simulink model "simpleModel"  (R2014b)
settings: Solver=ode45  StartTime=0.0  StopTime=10.0  RelTol=1e-3
settings Model: Creator=dmeissne  LastModifiedBy=dmeissne

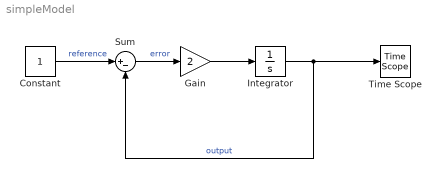
== system simpleModel ==
  Constant : Constant
  Gain : Gain  Gain=2
  Integrator : Integrator
  Sum : Sum  Inputs=|+-
  Time Scope : TimeScope  DefaultConfigurationName=spbscopes.TimeScopeBlockCfg
  wires:
  Integrator/1 -> Sum/2, Time Scope/1  "output"
  Constant/1 -> Sum/1  "reference"
  Sum/1 -> Gain/1  "error"
  Gain/1 -> Integrator/1
